simulink model "PID_values"  (R2017b)
settings: Solver=VariableStepAuto  StartTime=0.0  StopTime=20  RelTol=1e-3
undefined symbols (not defined in the file): T, tau, X
settings Model: Creator=Usuario  LastModifiedBy=Usuario

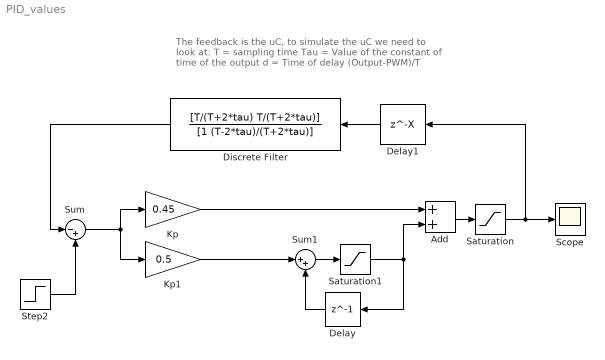
== system PID_values ==
  note: The feedback is the uC, to simulate the uC we need to
      | look at:
      | T = sampling time
      | Tau = Value of the constant of time of the output
      | d = Time of delay (Output-PWM)/T
  Add : Sum
  Delay : Delay  DelayLength=1
  Delay1 : Delay  DelayLength=X
  Discrete Filter : DiscreteFilter  Numerator=[T/(T+2*tau) T/(T+2*tau)]  Denominator=[1 (T-2*tau)/(T+2*tau)]
  Kp : Gain  Gain=0.45
  Kp1 : Gain  Gain=0.5
  Saturation : Saturate
  Saturation1 : Saturate
  Scope : Scope
  Step2 : Step  Time=0.1  After=255  SampleTime=0
  Sum : Sum  Inputs=|-+
  Sum1 : Sum  Inputs=|++
  wires:
  Step2/1 -> Sum/2
  Sum/1 -> Kp/1, Kp1/1
  Kp/1 -> Add/1
  Kp1/1 -> Sum1/1
  Delay/1 -> Sum1/2
  Discrete Filter/1 -> Sum/1
  Add/1 -> Saturation/1
  Sum1/1 -> Saturation1/1
  Delay1/1 -> Discrete Filter/1
  Saturation/1 -> Delay1/1, Scope/1
  Saturation1/1 -> Delay/1, Add/2
